simulink model "VarabeiFirsttask"  (R2016a)
settings: Solver=VariableStepAuto  StartTime=0.0  StopTime=10.0  RelTol=1e-3
libraries: simulink x1
settings Model: Creator=Student  LastModifiedBy=Student

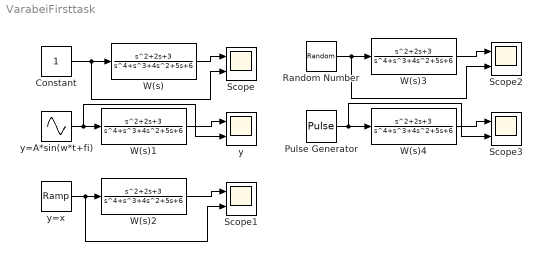
== system VarabeiFirsttask ==
  Constant : Constant
  Pulse Generator : DiscretePulseGenerator  PulseType=Time based  Period=3  PulseWidth=5
  Random Number : RandomNumber  SampleTime=0.1
  Scope{,1..3} (4 alike) : Scope  NumInputPorts=2
  W(s){,1..4} (5 alike) : TransferFcn  Numerator=[1 2 3]  Denominator=[1 1 4 5 6]
  y : Scope  NumInputPorts=2
  y=A*sin(w*t+fi) : Sin  SampleTime=0
  y=x : simulink/Sources/Ramp  slope=1  start=0  X0=0
  wires:
  y=A*sin(w*t+fi)/1 -> y/2, W(s)1/1
  y=x/1 -> Scope1/2, W(s)2/1
  Pulse Generator/1 -> Scope3/2, W(s)4/1
  W(s)/1 -> Scope/1
  Constant/1 -> Scope/2, W(s)/1
  W(s)1/1 -> y/1
  W(s)2/1 -> Scope1/1
  W(s)3/1 -> Scope2/1
  W(s)4/1 -> Scope3/1
  Random Number/1 -> Scope2/2, W(s)3/1
